simulink model "A_search"  (R2021b)
settings: Solver=ode1  StartTime=0.0  StopTime=inf  FixedStep=10  RelTol=1e-3
libraries: TcTargetLib x8
settings Model: Creator=ATLabor  LastModifiedBy=ATLabor
settings OptimizationCC: DefaultParameterBehavior=Inlined  LocalBlockOutputs=off
settings RTWCC: Description=TwinCAT GRT Target  SystemTargetFile=TwinCatGrt.tlc  GenCodeOnly=on  TemplateMakefile=tcgrt_msbuild.tmf  TargetLang=C++
settings STFCustomTargetCC: TargetLangStandard=C++11 (ISO)  CombineOutputUpdateFcns=on  CodeInterfacePackaging=Reusable function  CPPClassGenCompliant=on  GRTInterface=off  GenerateAllocFcn=on  SystemTargetFile=TwinCatGrt.tlc
settings GRTTargetCC: TargetLangStandard=C++11 (ISO)  ParMdlRefBuildCompliant=off  CompOptLevelCompliant=off  ConcurrentExecutionCompliant=off  MatFileLogging=off  CodeInterfacePackaging=Reusable function  GenerateAllocFcn=on  UseToolchainInfoCompliant=off  ExtModeMexFile=TcExtModeClient

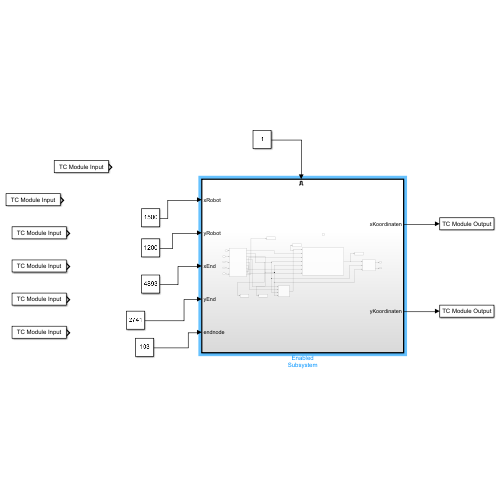
[thumbnail: Simulink's stored preview of the top-level diagram]
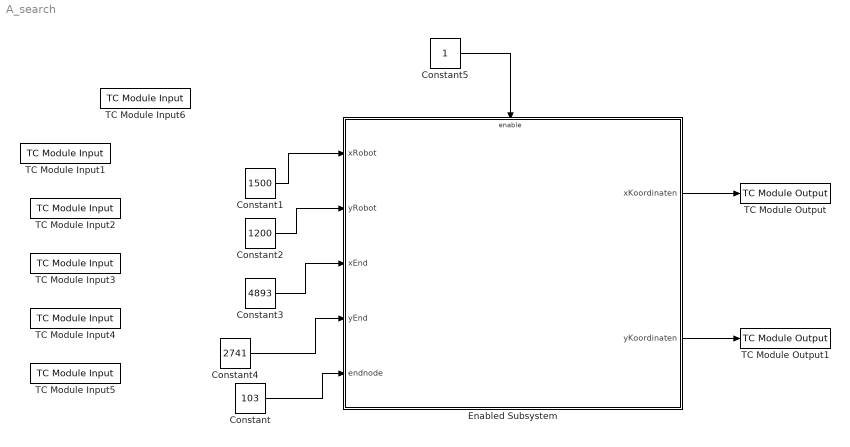
== system A_search ==
  Constant : Constant  Value=103
  Constant1 : Constant  Value=1500
  Constant2 : Constant  Value=1200
  Constant3 : Constant  Value=4893
  Constant4 : Constant  Value=2741
  Constant5 : Constant
  Enabled Subsystem : Subsystem  TreatAsAtomicUnit=on
  TC Module Input{1..6} (6 alike) : TcTargetLib/TC Module Input  PortDataType=double  PortDim=1  Value=0  SampleTime=-1  CodeGenConnectType=DataArea (InputDst)  DataTypeOverride=off
      settings: SourceProductName=Beckhoff TwinCAT Target
  TC Module Output : TcTargetLib/TC Module Output  PortDataType=double  PortDim=144:1  SampleTime=-1  CodeGenConnectType=DataArea (OutputSrc)  DataTypeOverride=off
      settings: SourceProductName=Beckhoff TwinCAT Target
  TC Module Output1 : TcTargetLib/TC Module Output  PortDataType=double  PortDim=144:1  SampleTime=-1  CodeGenConnectType=DataArea (OutputSrc)  DataTypeOverride=off
      settings: SourceProductName=Beckhoff TwinCAT Target
  wires:
  Enabled Subsystem/1(xKoordinaten) -> TC Module Output/1
  Enabled Subsystem/2(yKoordinaten) -> TC Module Output1/1
  Constant/1 -> Enabled Subsystem/5(endnode)
  Constant1/1 -> Enabled Subsystem/1(xRobot)
  Constant2/1 -> Enabled Subsystem/2(yRobot)
  Constant3/1 -> Enabled Subsystem/3(xEnd)
  Constant4/1 -> Enabled Subsystem/4(yEnd)
  Constant5/1 -> Enabled Subsystem/Enable

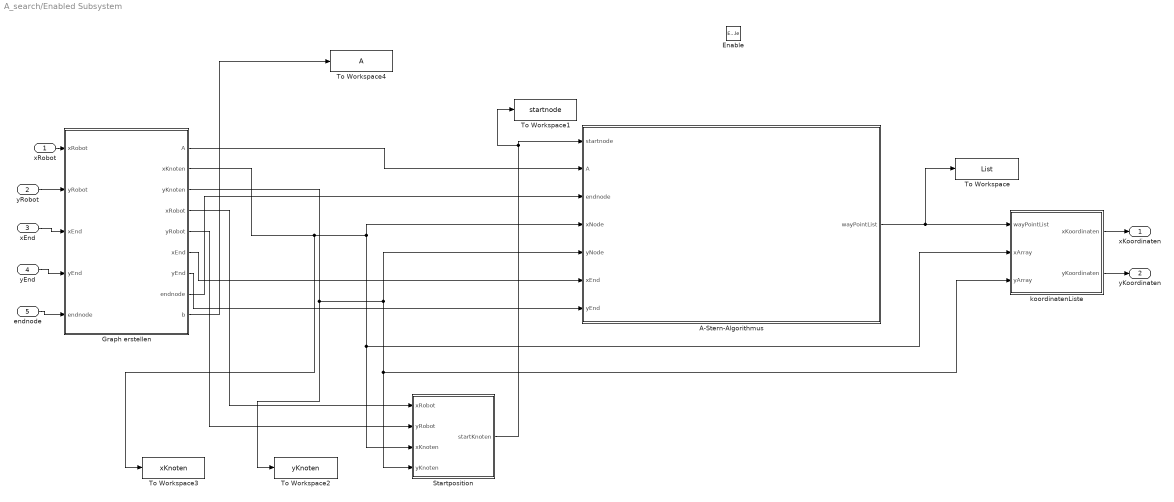
== system A_search/Enabled Subsystem ==
  xRobot : Inport
  yRobot : Inport  Port=2
  xEnd : Inport  Port=3
  yEnd : Inport  Port=4
  endnode : Inport  Port=5
  Enable : EnablePort
  A-Stern-Algorithmus : MATLAB Function  TreatAsAtomicUnit=on
  Graph erstellen : MATLAB Function  TreatAsAtomicUnit=on
  Startposition : MATLAB Function  TreatAsAtomicUnit=on
  To Workspace : ToWorkspace  VariableName=List  SampleTime=-1
  To Workspace1 : ToWorkspace  VariableName=startnode  SampleTime=-1
  To Workspace2 : ToWorkspace  VariableName=yKnoten  SampleTime=-1
  To Workspace3 : ToWorkspace  VariableName=xKnoten  SampleTime=-1
  To Workspace4 : ToWorkspace  VariableName=A  SampleTime=-1
      settings: Save2DSignal=2-D array (concatenate along first dimension)
  koordinatenListe : MATLAB Function  TreatAsAtomicUnit=on
  xKoordinaten : Outport
  yKoordinaten : Outport  Port=2
  wires:
  Graph erstellen/2(xKnoten) -> To Workspace3/1, A-Stern-Algorithmus/4(xNode), koordinatenListe/2(xArray), Startposition/3(xKnoten)
  koordinatenListe/1(xKoordinaten) -> xKoordinaten/1
  koordinatenListe/2(yKoordinaten) -> yKoordinaten/1
  Startposition/1(startKnoten) -> To Workspace1/1, A-Stern-Algorithmus/1(startnode)
  Graph erstellen/3(yKnoten) -> To Workspace2/1, koordinatenListe/3(yArray), Startposition/4(yKnoten), A-Stern-Algorithmus/5(yNode)
  Graph erstellen/1(A) -> A-Stern-Algorithmus/2(A)
  A-Stern-Algorithmus/1(wayPointList) -> To Workspace/1, koordinatenListe/1(wayPointList)
  endnode/1 -> Graph erstellen/5("endnode ")
  Graph erstellen/8(endnode) -> A-Stern-Algorithmus/3(endnode)
  yEnd/1 -> Graph erstellen/4("yEnd ")
  xEnd/1 -> Graph erstellen/3("xEnd ")
  Graph erstellen/6(xEnd) -> A-Stern-Algorithmus/6(xEnd)
  Graph erstellen/7(yEnd) -> A-Stern-Algorithmus/7(yEnd)
  xRobot/1 -> Graph erstellen/1("xRobot ")
  yRobot/1 -> Graph erstellen/2("yRobot ")
  Graph erstellen/5(yRobot) -> Startposition/2(yRobot)
  Graph erstellen/4(xRobot) -> Startposition/1(xRobot)
  Graph erstellen/9(b) -> To Workspace4/1

== matlab function A_search/Enabled Subsystem/Graph erstellen ==
  data: xRobot input; yRobot input; xEnd input; yEnd input; A output; xKnoten output; yKnoten output; xRobot output; yRobot output; xEnd output; yEnd output; endnode input; endnode output; b output
function [A, xKnoten, yKnoten, xRobot, yRobot, xEnd, yEnd, endnode, b]= fcn(xRobot, yRobot, xEnd, yEnd,endnode)

numberOfNodes = 144;
numberOfColumns = 18;
A = zeros(numberOfNodes);

% Verbindung zu relevanten Knoten
for i = 1:numberOfNodes
    if i-1>0 && mod(i, numberOfColumns) ~= 1
        A(i-1,i) = 1000;
    end
    if i+1<numberOfNodes+1 && mod(i,numberOfColumns) ~= 0
        A(i+1,i)= 1000;
    end
    if i+numberOfColumns<numberOfNodes+1
        A(i+numberOfColumns,i)=1000;
    end
    if i-numberOfColumns>0
        A(i-numberOfColumns,i)=1000;
    end
    if i+numberOfColumns+1 < numberOfNodes+1 && mod(i,numberOfColumns) ~= 0
        A(i+numberOfColumns+1,i) = sqrt(2)*1000;
    end
    if i+numberOfColumns-1 < numberOfNodes+1 && mod(i, numberOfColumns) ~= 1
        A(i+numberOfColumns-1,i) = sqrt(2)*1000;
    end
     if i-numberOfColumns+1 > 0 && mod(i,numberOfColumns) ~= 1
        A(i-numberOfColumns+1,i) = sqrt(2)*1000;
    end
    if i-numberOfColumns-1 > 0 && mod(i, numberOfColumns) ~= 0
        A(i-numberOfColumns-1,i) = sqrt(2)*1000;
    end
end

% Lösen der Station
for i= 1:144
    A(92,i) = 0;
    A(i,92) = 0;
    A(93,i) = 0;
    A(i,93) = 0;
    A(96,i) = 0;
    A(i,96) = 0;
    A(99,i) = 0;
    A(i,99) = 0;
    A(102,i) = 0;
    A(i,102) = 0;
    A(110,i) = 0;
    A(i,110) = 0;
    A(111,i) = 0;
    A(i,111) = 0;
    A(114,i) = 0;
    A(i,114) = 0;
    A(117,i) = 0;
    A(i,117) = 0;
    A(120,i) = 0;
    A(i,120) = 0;
    A(124,i) = 0;
    A(i,124) = 0;
    A(125,i) = 0;
    A(i,125) = 0;
    A(142,i) = 0;
    A(i,142) = 0;
    A(143,i) = 0;
    A(i,143) = 0;
end

%Graph = graph(A);

% Umrechung von Knoten in Koordinaten
xKnoten = zeros(numberOfNodes,1);
yKnoten = zeros(numberOfNodes,1);
row = 600;
col = 200;
for i = 1:numberOfNodes
    xKnoten(i) = col;
    yKnoten(i) = row;
    col = col + 400;
    if mod(i,numberOfColumns) == 0 
        col = 200;
        row = row + 400;
    end 
end

b = 2;

== matlab function A_search/Enabled Subsystem/A-Stern-Algorithmus ==
  data: startnode input; wayPointList output; A input; endnode input; xNode input; yNode input; xEnd input; yEnd input
function wayPointList = fcn(startnode, A, endnode, xNode, yNode, xEnd, yEnd)

Graph = graph(A);

%remoove nodes
%Graph = rmnode(Graph, [...]) 
numberOfNodes = 144;
%h = [7; 6; 5; 4; 6; 5; 4; 3; 5; 4; 3; 2; 4; 3; 2; 1; 3; 2; 1; 0];

openList = zeros(50,5);         % 1: Node, 2: f, 3: g, 4: ParentNode, 5: h
openList(1,1) = startnode;
closedList = zeros(50,4);       % 1: Node, 2: f, 3: g, 4: ParentNode, 5: h
f = sqrt(power(xNode(startnode)-xEnd,2) + power(yNode(startnode)-yEnd,2)); 
% weil f = g + h und g müsste bei Startknoten 0 sein
openList(1,2) = f;
g = zeros(numberOfNodes,1);
g(startnode) = 0;
openList(1,3) = g(startnode);
gParent = 0;
counter = 1;
nextNode = startnode;
actualNode = 0;
inClosedList = false;
inOpenList = false;

while (nextNode ~= endnode)
    
%Suche nach Node mit kleinstem f in openList
    for i = 1:numberOfNodes % alle Knoten aus openList durchgehen und kleinstes f(n) suchen
        if openList(i,1)~=0
            actualNode = openList(i,1);
        else
            break;
        end

        if actualNode > 1
            row1 = outedges(Graph,nextNode); % alle Zeilen in G (von Kanten) wo Knoten 6 beteiligt ist
            row2 = outedges(Graph,actualNode); % alle Zeilen in G wo aktueller Knoten beteiligt ist
            searchedRow = intersect(row1,row2);
            if openList(i,2) == 0
                g(actualNode) = gParent + Graph.Edges.Weight(searchedRow); %Gewichtung von Knoten in openList
                h = sqrt(power(xNode(actualNode)-xEnd,2) + power(yNode(actualNode)-yEnd,2));
                f = g(actualNode) + h(actualNode);
                openList(i,2) = f;
                openList(i,5) = h;
            end
        end
    end
    % Node mit kleinstem f finden
    if actualNode > 1
        Z=openList(:,2);
        Z(Z==0)=nan;
        fmin = min(Z);
        index = find(openList(:,2)==fmin);
        nextNode = openList(index(1),1);
        gParent = g(nextNode);
    else
        fmin = 0;
        nextNode = startnode;
        gParent = 0;
    end

 % Endknoten erreicht?
    if nextNode == endnode
        break;
    end
  
% nächstes Node in closed List einfügen und in openList löschen
    closedList(counter,1) = nextNode;
    closedList(counter,2) = fmin;
    closedList(counter,3) = gParent;
    if counter > 1
        closedList(counter,4) = closedList(counter-1,1);
    end
    openList = zeros(50,5);
    counter = counter + 1;

 % Nachbarn suchen und openList hinzufügen
    neighborsArray = neighbors(Graph,nextNode);
    neighborsRow = outedges(Graph,nextNode);
    for n = 1:length(neighborsArray)
        actualNeighbor = neighborsArray(n);
        gNeighbor = gParent + Graph.Edges.Weight(neighborsRow(n));
        for index = 1:size(closedList,1)
            if closedList(index,1) == actualNeighbor
                inClosedList = true;
            end
             if openList(index,1) == actualNeighbor
                inOpenList = true;
             end
        end

        if gNeighbor < gParent  && inClosedList == true
            closedList(closedList(:,1)==actualNeighbor,3) = gNeighbor;
            closedList(closedList(:,1)==actualNeighbor,4) = nextNode;
        elseif gNeighbor < gParent && inOpenList == true
                openList(openList(:,1)==actualNeighbor,3) = gNeighbor;
                openList(openList(:,1)==actualNeighbor,4) = nextNode;         
        elseif inClosedList == false && inOpenList == false
                    nextIndex = find(openList(:,1)==0);
                    openList(nextIndex(1),1) = actualNeighbor;
                    openList(nextIndex(1),3) = gNeighbor;
        end
        inClosedList = false;
        inOpenList = false;
    end
end

closedList(counter,1) = endnode;
wayPointList = zeros(20,1);
for index = 1:counter
    wayPointList(index) = closedList(index,1);
end

== matlab function A_search/Enabled Subsystem/Startposition ==
  data: xRobot input; startKnoten output; yRobot input; xKnoten input; yKnoten input
function startKnoten= fcn(xRobot, yRobot, xKnoten, yKnoten)

startKnoten = 0;
startKnotenArray = 0;
diff_x = zeros(size(xKnoten,1),1);
diff_y = zeros(size(yKnoten,1),1);

for i = 1:size(xKnoten,1)
    diff_x(i) = abs(xRobot-xKnoten(i));
end

for i = 1:size(yKnoten,1)
    diff_y(i) = abs(yRobot-yKnoten(i));
end

xMin = min(diff_x);
yMin = min(diff_y);

xStart = find(diff_x == xMin);
yStart = find(diff_y == yMin);

startKnotenArray = intersect(xStart, yStart);

startKnoten = startKnotenArray(1,1);

== matlab function A_search/Enabled Subsystem/koordinatenListe ==
  data: wayPointList input; xKoordinaten output; yKoordinaten output; xArray input; yArray input
function [xKoordinaten, yKoordinaten]= fcn(wayPointList, xArray, yArray)

sizeList = size(wayPointList,1);
xKoordinaten = zeros(sizeList,1);
yKoordinaten = zeros(sizeList,1);

for i = 1 : sizeList
    xKoordinaten(i) = xArray(wayPointList(i));
    yKoordinaten(i) = yArray(wayPointList(i));
end
